simulink model "pll_3"  (Simulink 2.20)
settings: Solver=ode45  StartTime=0.0  StopTime=10.0  RelTol=1e-3  AbsTol=1e-6
settings Model: ConsistencyChecking=off  RTWPlaceOutputsASAP=off

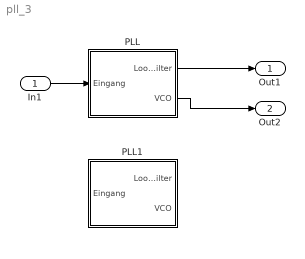
== system pll_3 ==
  In1 : Inport  Port=1  PortWidth=-1  SampleTime=-1
  PLL : Subsystem
  PLL1 : Subsystem
  Out1 : Outport  Port=1
  Out2 : Outport  Port=2
  wires:
  In1/1 -> PLL/1(Eingang)
  PLL/1(Loop-Filter) -> Out1/1
  PLL/2(" VCO") -> Out2/1

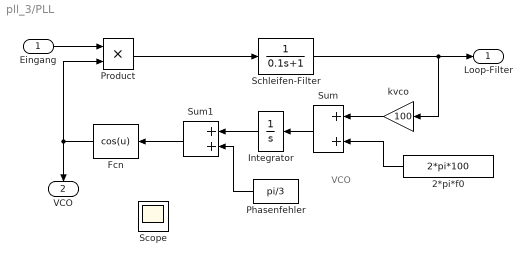
== system pll_3/PLL ==
  note: VCO
  Eingang : Inport  Port=1  PortWidth=-1  SampleTime=-1
  2*pi*f0 : Constant  Orientation=left  Value=2*pi*100
  Fcn : Fcn  Orientation=left  Expr=cos(u)
  Integrator : Integrator  Orientation=left  ExternalReset=none  InitialConditionSource=internal  InitialCondition=0  LimitOutput=off  UpperSaturationLimit=inf  LowerSaturationLimit=-inf  ShowSaturationPort=off  ShowStatePort=off  AbsoluteTolerance=auto
  Phasenfehler : Constant  Orientation=left  Value=pi/3
  Product : Product  Inputs=2
  Schleifen-Filter : TransferFcn  Numerator=[1]  Denominator=[0.1 1]
  Scope : Scope
      settings: Floating=on  TickLabels=on  TimeRange=0.1  YMin=-5  YMax=5  SaveToWorkspace=off  SaveName=ScopeData
  Sum : Sum  Orientation=left  Inputs=++
  Sum1 : Sum  Orientation=left  Inputs=++
  kvco : Gain  Orientation=left  Gain=100
  Loop-Filter : Outport  Port=1  InitialOutput=0
  " VCO" : Outport  Orientation=down  Port=2  InitialOutput=0
  wires:
  Integrator/1 -> Sum1/1
  Phasenfehler/1 -> Sum1/2
  Schleifen-Filter/1 -> Loop-Filter/1, kvco/1
  kvco/1 -> Sum/1
  2*pi*f0/1 -> Sum/2
  Sum/1 -> Integrator/1
  Product/1 -> Schleifen-Filter/1
  Sum1/1 -> Fcn/1
  Eingang/1 -> Product/1
  Fcn/1 -> " VCO"/1, Product/2

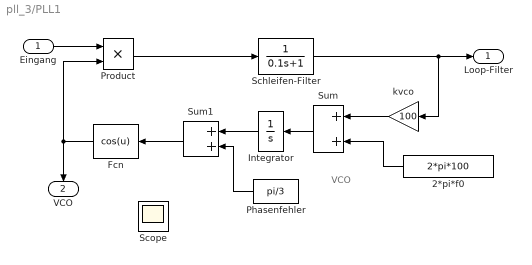
== system pll_3/PLL1 ==
  note: VCO
  Eingang : Inport  Port=1  PortWidth=-1  SampleTime=-1
  2*pi*f0 : Constant  Orientation=left  Value=2*pi*100
  Fcn : Fcn  Orientation=left  Expr=cos(u)
  Integrator : Integrator  Orientation=left  ExternalReset=none  InitialConditionSource=internal  InitialCondition=0  LimitOutput=off  UpperSaturationLimit=inf  LowerSaturationLimit=-inf  ShowSaturationPort=off  ShowStatePort=off  AbsoluteTolerance=auto
  Phasenfehler : Constant  Orientation=left  Value=pi/3
  Product : Product  Inputs=2
  Schleifen-Filter : TransferFcn  Numerator=[1]  Denominator=[0.1 1]
  Scope : Scope
      settings: Floating=on  TickLabels=on  TimeRange=0.1  YMin=-5  YMax=5  SaveToWorkspace=off  SaveName=ScopeData
  Sum : Sum  Orientation=left  Inputs=++
  Sum1 : Sum  Orientation=left  Inputs=++
  kvco : Gain  Orientation=left  Gain=100
  Loop-Filter : Outport  Port=1  InitialOutput=0
  " VCO" : Outport  Orientation=down  Port=2  InitialOutput=0
  wires:
  Fcn/1 -> Product/2, " VCO"/1
  Eingang/1 -> Product/1
  Sum1/1 -> Fcn/1
  Product/1 -> Schleifen-Filter/1
  Sum/1 -> Integrator/1
  2*pi*f0/1 -> Sum/2
  kvco/1 -> Sum/1
  Schleifen-Filter/1 -> kvco/1, Loop-Filter/1
  Phasenfehler/1 -> Sum1/2
  Integrator/1 -> Sum1/1
